simulink model "F16_Longitude"  (R2021a)
settings: Solver=VariableStepAuto  StartTime=0.0  StopTime=300  RelTol=1e-3
values from neighbouring files (symbols this model uses):
  A_longitude_lo = sel(mat_lo,[1 3 5 8 13], [1 3 5 8 13])    [FindF16Dynamics.m]
  B_longitude_lo = sel(mat_lo,[1 3 5 8 13], [14 15])    [FindF16Dynamics.m]
  C_longitude_lo = sel(mat_lo,[14 16 18 21 26], [1 3 5 8 13])    [FindF16Dynamics.m]
  D_longitude_lo = sel(mat_lo,[14 16 18 21 26], [14 15])    [FindF16Dynamics.m]
settings Model: Creator=LXS  LastModifiedBy=Goodluck
settings SolverCC: AlgebraicLoopSolver=TrustRegion
settings DataIOCC: ReturnWorkspaceOutputs=off
settings DebuggingCC: SFMachineParentedDataDiag=warning  ArithmeticOperatorsInVariantConditions=warning
settings SFSimCC: CustomCodeUndefinedFunction=UseInterfaceOnly

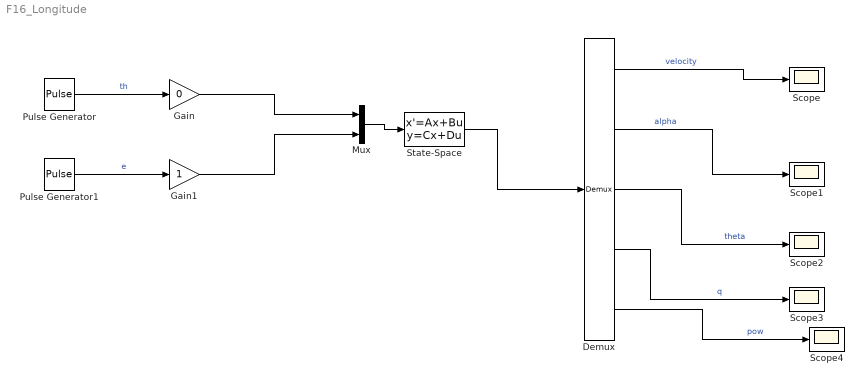
== system F16_Longitude ==
  Demux : Demux  Outputs=5
  Gain : Gain  Gain=0
  Gain1 : Gain
  Mux : Mux  Inputs=2
  Pulse Generator : DiscretePulseGenerator  PulseType=Time based  Period=0.1
  Pulse Generator1 : DiscretePulseGenerator  PulseType=Time based  Amplitude=0.01  Period=300
  Scope{,1..4} (5 alike) : Scope
  State-Space : StateSpace  A=A_longitude_lo  B=B_longitude_lo  C=C_longitude_lo  D=D_longitude_lo  InitialCondition=0
  wires:
  State-Space/1 -> Demux/1
  Demux/1 -> Scope/1  "velocity"
  Demux/2 -> Scope1/1  "alpha"
  Demux/3 -> Scope2/1  "theta"
  Demux/4 -> Scope3/1  "q"
  Pulse Generator/1 -> Gain/1  "th"
  Pulse Generator1/1 -> Gain1/1  "e"
  Mux/1 -> State-Space/1
  Gain/1 -> Mux/1
  Gain1/1 -> Mux/2
  Demux/5 -> Scope4/1  "pow"
